simulink model "Motor_Diesel_paC2"  (R2017a)
settings: Solver=VariableStepAuto  StartTime=0.0  StopTime=1  RelTol=1e-3  EnableMultiTasking=on
values from neighbouring files (symbols this model uses):
  H_act_d = c2d (H_act, 0.01,'tustin')    [InicC.m]
  K1 = 1.15    [InicC.m]
settings Model: Creator=dmartinez  LastModifiedBy=Administrador
settings OptimizationCC: LifeSpan=inf
settings DebuggingCC: SFUnexpectedBacktrackingDiag=warning  SFNoUnconditionalDefaultTransitionDiag=warning  SFExecutionAtInitializationDiag=none
settings GRTTargetCC: TargetLangStandard=C89/C90 (ANSI)  GeneratePreprocessorConditionals=Disable all
settings ConfigComp: CovMetricSettings=dw  CovHtmlReporting=on  CovSaveCumulativeToWorkspaceVar=on  CovSaveSingleToWorkspaceVar=on  CovExternalEMLEnable=off

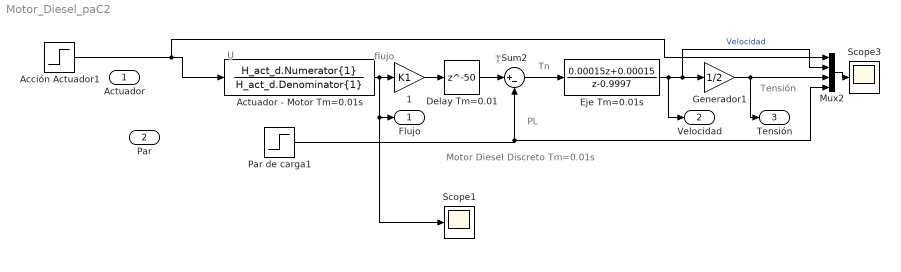
== system Motor_Diesel_paC2 ==
  note: flujo
  note: T
  note: U
  note: PL
  note: Tn
  note: Motor Diesel Discreto Tm=0.01s
  note: Tensión
  Actuador : Inport
  Par : Inport  Port=2
  " 1" : Gain  Gain=K1
  " Generador1" : Gain  Gain=1/2
  Acción Actuador1 : Step  Time=0  SampleTime=0
  Actuador - Motor Tm=0.01s : DiscreteTransferFcn  Numerator=H_act_d.Numerator{1}  Denominator=H_act_d.Denominator{1}  SampleTime=0.01
  Delay Tm=0.01 : Delay  DelayLength=50  SampleTime=0.01
  Eje Tm=0.01s : DiscreteTransferFcn  Numerator=[0.00015 0.00015]  Denominator=[1 -0.9997]  SampleTime=0.01
  Mux2 : Mux
  Par de carga1 : Step  Time=300  Before=0.1  SampleTime=0
  Scope1 : Scope
  Scope3 : Scope
  Sum2 : Sum  Inputs=|+-
  Flujo : Outport
  Velocidad : Outport  Port=2
  Tensión : Outport  Port=3
  wires:
  Mux2/1 -> Scope3/1
  Sum2/1 -> Eje Tm=0.01s/1
  Eje Tm=0.01s/1 -> Velocidad/1, Mux2/2, " Generador1"/1  "Velocidad"
  " Generador1"/1 -> Tensión/1, Mux2/3
  Actuador - Motor Tm=0.01s/1 -> Scope1/1, Flujo/1, " 1"/1
  " 1"/1 -> Delay Tm=0.01/1
  Delay Tm=0.01/1 -> Sum2/1
  Acción Actuador1/1 -> Mux2/1, Actuador - Motor Tm=0.01s/1
  Par de carga1/1 -> Mux2/4, Sum2/2
